simulink model "my_demo_ref2"  (R2012b)
settings: Solver=FixedStepDiscrete  StartTime=0.0  StopTime=Inf  FixedStep=0.033  RelTol=1e-3
values from neighbouring files (symbols this model uses):
  fpath = [mypath(2:length(mypath),:); lin; pf]    [robot_path.m]
undefined symbols (not defined in the file or in its folder): magnitude
libraries: simiam x5, vrlib x1, simulink x1
settings Model: Creator=jdelacroix  LastModifiedBy=samati
settings DataIOCC: SignalLoggingSaveFormat=ModelDataLogs  SaveOutput=off  SaveTime=off
settings DebuggingCC: MultiTaskDSMMsg=warning  MultiTaskCondExecSysMsg=none  FcnCallInpInsideContextMsg=EnableAllAsWarning  StrictBusMsg=None
settings RTWCC: IncludeERTFirstTime=on
settings CodeAppCC: CustomSymbolStrType=$N$R$M_T  InternalIdentifier=Shortened
settings GRTTargetCC: CodeReplacementLibrary=None  CPPClassGenCompliant=on

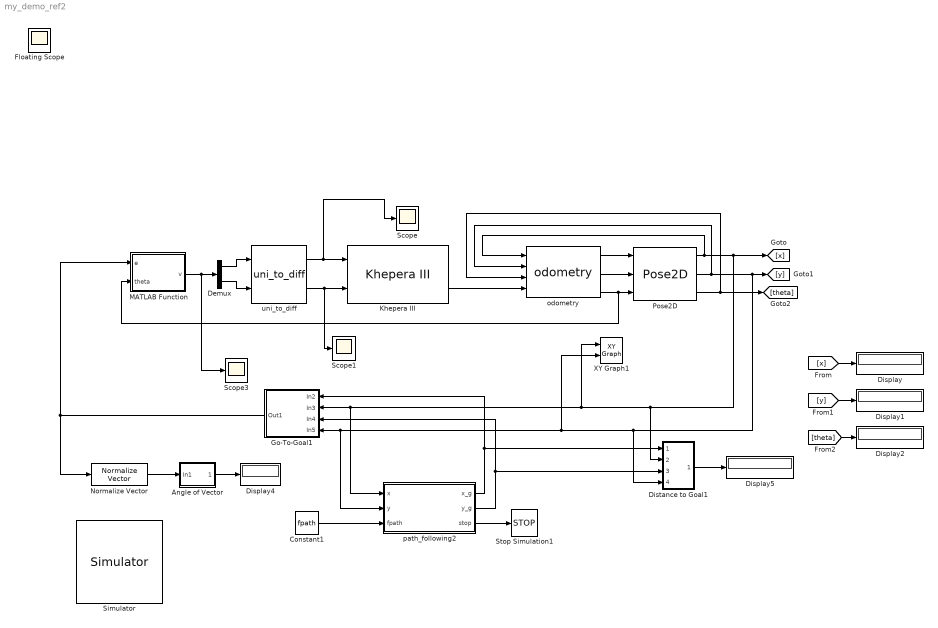
== system my_demo_ref2 ==
  Angle of Vector : Subsystem
      mask Display:
      | port_label('input', 1, 'u')
      | port_label('output', 1, 'theta')
  Constant1 : Constant  Value=fpath
  Demux : Demux  Outputs=2
  Display{,1..2,4..5} (5 alike) : Display
  Distance to Goal1 : Subsystem
      mask Display:
      | port_label('input', 1, 'x_g')
      | port_label('input', 2, 'x')
      | port_label('input', 3, 'y_g')
      | port_label('input', 4, 'y')
      | port_label('output', 1, 'd')
  Go-To-Goal1 : Subsystem
      mask Display:
      | port_label('input', 1, 'x_g')
      | port_label('input', 2, 'x')
      | port_label('input', 3, 'y_g')
      | port_label('input', 4, 'y')
      | port_label('output', 1, 'u_gtg')
  Khepera III : simiam/Khepera III  x_0=xi  y_0=yi  theta_0=thetai  robot_id=1
  MATLAB Function : MATLAB Function  TreatAsAtomicUnit=on
  Normalize Vector : vrlib/Utilities/Normalize Vector  maxzero=0
  Pose2D : simiam/Pose2D  SystemSampleTime=-1
  Scope : Scope
  Scope1 : Scope
      settings: SaveName=ScopeData2
  Scope3 : Scope
      settings: YMin=-3.5  YMax=1  SaveName=ScopeData4
  Simulator : simiam/Simulator  Priority=1
  Stop Simulation1 : Stop
  XY Graph1 : simulink/Sinks/XY Graph  xmin=-3  xmax=3  ymin=-3  ymax=3  st=-1
  odometry : simiam/odometry  wheel_radius=r  wheel_base_length=l  ticks_per_rev=ticks
  "path_following2 " : MATLAB Function  TreatAsAtomicUnit=on
  uni_to_diff : simiam/uni_to_diff  wheel_radius=r  wheel_base_length=l
  Floating Scope : Scope
      settings: Floating=on
  wires:
  uni_to_diff/1 -> Scope/1, Khepera III/1
  odometry/3 -> MATLAB Function/2(theta), Pose2D/3
  odometry/2 -> Pose2D/2
  odometry/1 -> Pose2D/1
  Khepera III/2 -> odometry/4
  Go-To-Goal1/1(Out1) -> MATLAB Function/1(e), Normalize Vector/1
  Pose2D/3 -> [theta], odometry/3
  Normalize Vector/1 -> Angle of Vector/1(In1)
  Angle of Vector/1(Out1) -> Display4/1
  Demux/1 -> uni_to_diff/1
  Demux/2 -> uni_to_diff/2
  MATLAB Function/1(v) -> Scope3/1, Demux/1
  Pose2D/1 -> Distance to Goal1/2(In2), XY Graph1/1, Go-To-Goal1/2(In3), "path_following2 "/1(x), [x], odometry/1
  Pose2D/2 -> Distance to Goal1/4(In4), XY Graph1/2, Go-To-Goal1/4(In5), "path_following2 "/2(y), [y], odometry/2
  [theta] -> Display2/1
  [y] -> Display1/1
  "path_following2 "/1(x_g) -> Distance to Goal1/1(In1), Go-To-Goal1/1(In2)
  "path_following2 "/2(y_g) -> Distance to Goal1/3(In3), Go-To-Goal1/3(In4)
  Constant1/1 -> "path_following2 "/3(fpath)
  "path_following2 "/3(stop) -> Stop Simulation1/1
  Distance to Goal1/1(Out1) -> Display5/1
  uni_to_diff/2 -> Scope1/1, Khepera III/2
  [x] -> Display/1

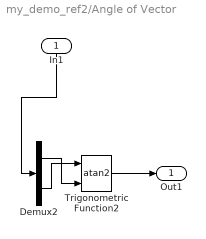
== system my_demo_ref2/Angle of Vector ==
  In1 : Inport
  Demux2 : Demux  Outputs=2
  Trigonometric Function2 : Trigonometry  Operator=atan2
  Out1 : Outport
  wires:
  Trigonometric Function2/1 -> Out1/1
  Demux2/1 -> Trigonometric Function2/2
  Demux2/2 -> Trigonometric Function2/1
  In1/1 -> Demux2/1

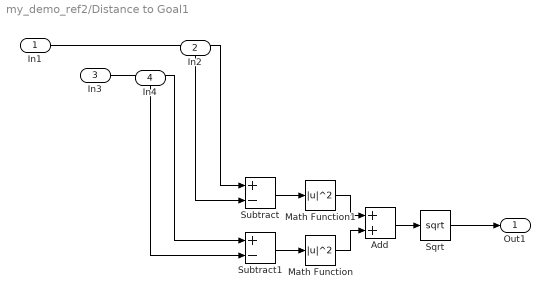
== system my_demo_ref2/Distance to Goal1 ==
  In1 : Inport
  In2 : Inport  Port=2
  In3 : Inport  Port=3
  In4 : Inport  Port=4
  Add : Sum
  Math Function : Math  Operator=magnitude^2  SaturateOnIntegerOverflow=on
  Math Function1 : Math  Operator=magnitude^2  SaturateOnIntegerOverflow=on
  Sqrt : Sqrt  SaturateOnIntegerOverflow=on
  Subtract : Sum  Inputs=+-
  Subtract1 : Sum  Inputs=+-
  Out1 : Outport
  wires:
  In4/1 -> Subtract1/2
  Subtract1/1 -> Math Function/1
  Math Function/1 -> Add/2
  Sqrt/1 -> Out1/1
  Subtract/1 -> Math Function1/1
  Math Function1/1 -> Add/1
  Add/1 -> Sqrt/1
  In2/1 -> Subtract/2
  In3/1 -> Subtract1/1
  In1/1 -> Subtract/1

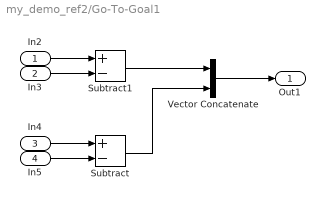
== system my_demo_ref2/Go-To-Goal1 ==
  In2 : Inport
  In3 : Inport  Port=2
  In4 : Inport  Port=3
  In5 : Inport  Port=4
  Subtract : Sum  Inputs=+-
  Subtract1 : Sum  Inputs=+-
  Vector Concatenate : Concatenate  Mode=Multidimensional array
  Out1 : Outport
  wires:
  In5/1 -> Subtract/2
  In2/1 -> Subtract1/1
  In3/1 -> Subtract1/2
  In4/1 -> Subtract/1
  Vector Concatenate/1 -> Out1/1
  Subtract1/1 -> Vector Concatenate/1
  Subtract/1 -> Vector Concatenate/2

== matlab function my_demo_ref2/MATLAB Function ==
  data: e input; v output; theta input
function v = fcn(e, theta)

l = 0.02;
mat = [1 0; 0 1/l];
R = [cos(-theta) -sin(-theta); sin(-theta) cos(-theta)];

u_max = 10;
a = 0.01;
k1 = 1./exp(abs(e(1))) + (u_max * (1-exp(-a.*e(1).^2))) ./ abs(e(1));
k2 = 1./exp(abs(e(2))) + (u_max * (1-exp(-a.*e(2).^2))) ./ abs(e(2));
K = [k1 0; 0 k2];

v = mat*R*K*e;

== matlab function my_demo_ref2/path_following2  ==
  data: x_g output; y_g output; x input; y input; fpath input; stop output
function [x_g, y_g, stop] = path_following2(x, y, fpath)
% PATH_FOLLOWINF Outputs next setpoint once the previous one has been 
% reached (from fpaht).

% Variables that need to stay from one call to another of the function
persistent i
if isempty(i)
   i = 1;
end

% Parameters
stop = 0;
dmin = 0.2;

% Set of points
% xx = [0.1 0.1 0.2 0.3 0.4 0.5 0.6 0.7 0.8 0.9 1];
% yy = [0.1 0.2 0.2 0.2 0.4 0.3 0.1 0.1 0.6 0.6 0.6];

% With pchip
% xxp = [0 1 2 3];
% yyp = [0 1 0 1.5];
% xx = 0:0.2:3;
% yy = pchip(xxp,yyp,xx);

% Check distant to current goal point to reach
xx = fpath(:,1);
yy = fpath(:,2);

d = sqrt((x-xx(i))^2 + (y-yy(i))^2);

if d < dmin && i < (length(xx))
    i = i + 1;
end

% Set new goal point 
x_g = xx(i);
y_g = yy(i);

% Give stop signal if last point was reached
if d < dmin && i == length(xx)
    stop = 1;
end

end
